simulink model "Second_Order_fixed_time_tracking_2014b"  (R2014a)
settings: Solver=ode4  StartTime=0.0  StopTime=20  FixedStep=0.001  RelTol=1e-3
settings Model: CovSFcnEnable=on  ExtModeTrigMode=oneshot  ExtModeArmWhenConnect=off  Creator=hp  LastModifiedBy=Administrator
settings DataIOCC: LimitDataPoints=off  SignalLoggingSaveFormat=ModelDataLogs  SignalLoggingName=sigsOut
settings OptimizationCC: BooleanDataType=off  ExpressionDepthLimit=2147483647  InitFltsAndDblsToZero=on
settings DebuggingCC: SaveWithParameterizedLinksMsg=none  UnderspecifiedInitializationDetection=Classic  SignalResolutionControl=TryResolveAllWithWarning  SolverPrmCheckMsg=none  MultiTaskDSMMsg=warning  MultiTaskCondExecSysMsg=none  FcnCallInpInsideContextMsg=EnableAllAsWarning  FrameProcessingCompatibilityMsg=error  StateNameClashWarn=warning
settings HardwareCC: TargetUnknown=on
settings GRTTargetCC: TargetFcnLib=ansi_tfl_tmw.mat  CombineOutputUpdateFcns=off  GRTInterface=on

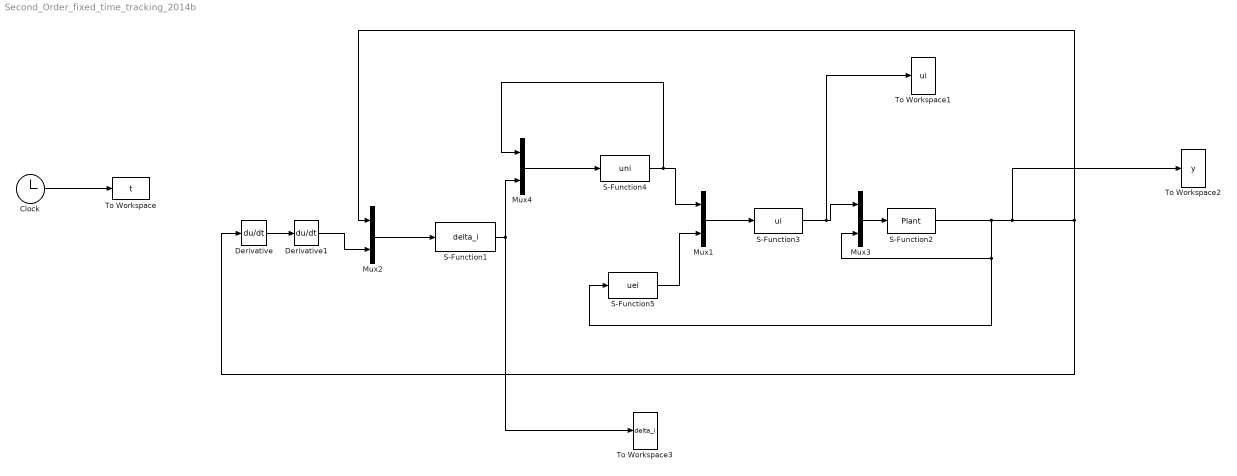
== system Second_Order_fixed_time_tracking_2014b ==
  Clock : Clock
  Derivative : Derivative
  Derivative1 : Derivative
  Mux{1..4} (4 alike) : Mux  Inputs=2
  S-Function1 : S-Function  FunctionName=delta_i  SFunctionDeploymentMode=off  EnableBusSupport=off
  S-Function2 : S-Function  FunctionName=Plant  SFunctionDeploymentMode=off  EnableBusSupport=off
  S-Function3 : S-Function  FunctionName=ui  SFunctionDeploymentMode=off  EnableBusSupport=off
  S-Function4 : S-Function  FunctionName=uni  SFunctionDeploymentMode=off  EnableBusSupport=off
  S-Function5 : S-Function  FunctionName=uei  SFunctionDeploymentMode=off  EnableBusSupport=off
  To Workspace : ToWorkspace  VariableName=t  SampleTime=-1
  To Workspace1 : ToWorkspace  VariableName=ui  SampleTime=-1
  To Workspace2 : ToWorkspace  VariableName=y  SampleTime=-1
  To Workspace3 : ToWorkspace  VariableName=delta_i  SampleTime=-1
  wires:
  Clock/1 -> To Workspace/1
  S-Function4/1 -> Mux4/1, Mux1/1
  S-Function5/1 -> Mux1/2
  Mux1/1 -> S-Function3/1
  Mux2/1 -> S-Function1/1
  S-Function2/1 -> Mux3/2, S-Function5/1, To Workspace2/1, Derivative/1, Mux2/1
  Mux4/1 -> S-Function4/1
  S-Function1/1 -> To Workspace3/1, Mux4/2
  Mux3/1 -> S-Function2/1
  S-Function3/1 -> To Workspace1/1, Mux3/1
  Derivative/1 -> Derivative1/1
  Derivative1/1 -> Mux2/2
